simulink model "AD_NOcontrolPIDposicionConObs_CompTermico_rampaPos_EscalVelo"  (R2012b)
settings: Solver=ode45  StartTime=0.0  StopTime=18  MaxStep=1e-4  RelTol=1e-4
values from neighbouring files (symbols this model uses):
  alfa_cu = 3.9*10^-3    (= 0.0039)    [InicializaYconstantes.m]
  b_m = bm+(bl/r^2)    (= 1.5e-05)    [InicializaYconstantes.m]
  Cts = 1.091    [InicializaYconstantes.m]
  J_m = Jm+(Jl/r^2)    (= 5.65099476805e-06)    [InicializaYconstantes.m]
  Kd = J_m*n*wpos    (= 0.0113019895361)    [InicializaYconstantes.m]
  Ketita = 2*3200-b_m/J_m    (= 6397.34560009)    [InicializaYconstantes.m]
  Kew = 3200^2-Ketita*b_m/J_m    (= 10223018.8864)    [InicializaYconstantes.m]
  Ki = J_m*wpos^3    (= 2893.30932124)    [InicializaYconstantes.m]
  Kp = J_m*n*wpos^2    (= 9.04159162887)    [InicializaYconstantes.m]
  lambda = 0.01546    [InicializaYconstantes.m]
  Ld = 6.6*10^-3    (= 0.0066)    [InicializaYconstantes.m]
  Lq = 5.8*10^-3    (= 0.0058)    [InicializaYconstantes.m]
  Pp = 3    [InicializaYconstantes.m]
  r = 314.3008    [InicializaYconstantes.m]
  R1 = -p1i*Lq    (= 29)    [InicializaYconstantes.m]
  R2 = -p1i*Ld    (= 33)    [InicializaYconstantes.m]
  Rs = 1.02    [InicializaYconstantes.m]
  Rs_cero = 1.02    [InicializaYconstantes.m]
  Rts = 55    [InicializaYconstantes.m]
  T_l = Tl/r    (= 0.00499521477515)    [InicializaYconstantes.m]
  Ta = 40    [InicializaYconstantes.m]
undefined symbols (not defined in the file or in its folder): sigbuilder_block
settings Model: Creator=usuario  LastModifiedBy=usuario

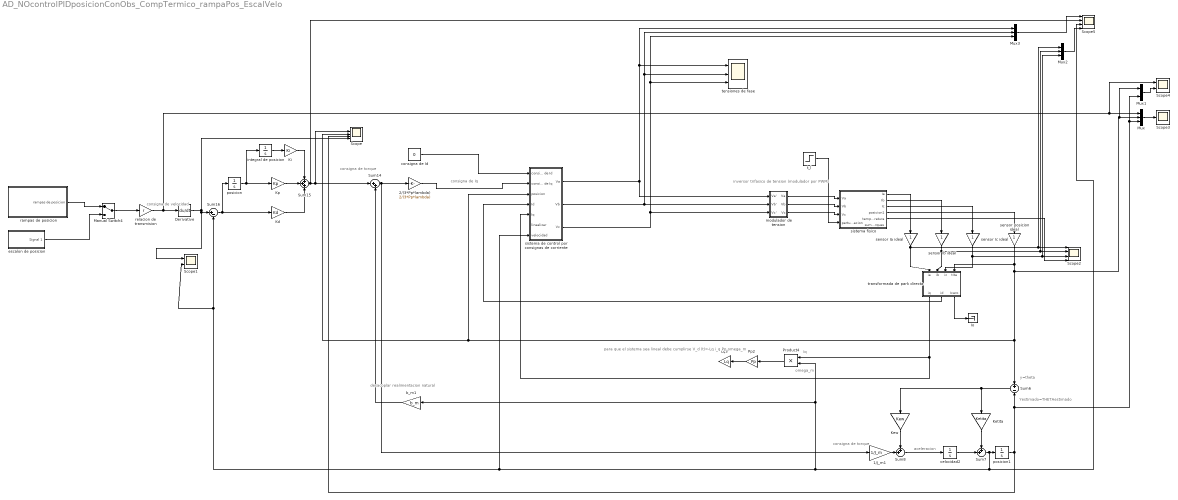
== system AD_NOcontrolPIDposicionConObs_CompTermico_rampaPos_EscalVelo ==
  note: consigna de velocidad
  note: aceleracion
  note: consigna de torque
  note: Yestimado=THETAestimado
  note: y=theta
  note: consigna de torque
  note: desacoplar
      | realimentacion natural
  note: consigna de Iq
  note: inversor trifasico de tension
      | (modulador por PWM)
  note: omega_m
  note: Iq
  note: para que el sistema sea lineal debe cumplirse
      | V_d (t)=-Lq  i_q  Pp omega_m
  1/J_m1 : Gain  Gain=1/J_m
  2/(3*Pp*lambda) : Gain  Gain=2/(3*Pp*lambda)
  Derivative : Derivative
  Io : Terminator
  Kd : Gain  Gain=Kd
  Ketita : Gain  Gain=Ketita
  Kew : Gain  Gain=Kew
  Ki : Gain  Gain=Ki
  Kp : Gain  Gain=Kp
  Lq3 : Gain  Gain=Lq
  Manual Switch4 : ManualSwitch
  Mux : Mux  Inputs=3
  Mux1 : Mux  Inputs=2
  Mux2 : Mux  Inputs=3
  Mux3 : Mux  Inputs=3
  Pp2 : Gain  Gain=Pp
  Product4 : Product  RndMeth=Zero
  Scope : Scope  NumInputPorts=5
      settings: TimeRange=10  YMin=2500~900~-400000~-400000~-2000  YMax=3200~1300~-200000~-200000~2000  SaveName=ScopeData5
  Scope1 : Scope  NumInputPorts=2
      settings: TimeRange=30  YMin=-5~-5.5  YMax=1~1  SaveName=ScopeData7
  Scope2 : Scope  NumInputPorts=4
      settings: YMin=-10~-50~-30~90  YMax=50~20~40~98  SaveName=ScopeData6
  Scope3 : Scope
      settings: TimeRange=10  YMin=-0.5  YMax=6  SaveName=ScopeData8
  Scope4 : Scope  NumInputPorts=2
      settings: TimeRange=10  YMin=-0.5~0  YMax=6~7  SaveName=ScopeData9
  Scope5 : Scope  NumInputPorts=4
      settings: YMin=-0.01~-0.08~-0.075~20  YMax=0.08~0.02~0.075~60  SaveName=ScopeData10
  Sum14 : Sum  Inputs=|++
  Sum15 : Sum  Inputs=+++
  Sum16 : Sum  Inputs=|+-
  Sum6 : Sum  Inputs=+-
  Sum7 : Sum  Inputs=++|
  Sum8 : Sum  Inputs=++|
  b_m1 : Gain  Gain=b_m
  consigna de Id : Constant  Value=0
  escalon de posicion : Subsystem  Tag=STV Subsys  LoadFcn=sigbuilder_block('load');  StartFcn=sigbuilder_block('start');  StopFcn=sigbuilder_block('stop');  ClipboardFcn=sigbuilder_block('clipboard');  mask(Sigbuilder block){}
      mask help: Simulink:masks:SigbuilderBlock_MD
      mask init:
      | if ~strcmp(get_param(bdroot(gcbh),'SimulationStatus'),'stopped') tuvar = sigbuilder_block('maskInit'); end
      settings: CopyFcn=sigbuilder_block('copy');  DeleteFcn=sigbuilder_block('delete');  ModelCloseFcn=sigbuilder_block('modelClose');  PreSaveFcn=sigbuilder_block('preSave');  PauseFcn=sigbuilder_block('pause');  ContinueFcn=sigbuilder_block('continue');  NameChangeFcn=sigbuilder_block('namechange');  OpenFcn=sigbuilder_block('open',[5.58621 27.931 836.69 391.034 ]);  CloseFcn=sigbuilder_block('close');
      mask Display: plot(0, 0, 100, 100,[2, 2, 32, 32, 2], [68, 8, 8, 68, 68],[32, 2], [38, 38], [32, 19, 2],[53, 60, 44], [32, 17, 17, 2],[16, 16, 31, 31]);txt = getActiveGroup(gcbh);text(2, 100, txt,'verticalAlignment', 'top');
  integral de posicion : Integrator
  modulador de tension : Subsystem
  posicion : Integrator
  posicion1 : Integrator
  rampas de posicion : Subsystem  Tag=STV Subsys  LoadFcn=sigbuilder_block('load');  StartFcn=sigbuilder_block('start');  StopFcn=sigbuilder_block('stop');  ClipboardFcn=sigbuilder_block('clipboard');  mask(Sigbuilder block){}
      mask help: Simulink:masks:SigbuilderBlock_MD
      mask init:
      | if ~strcmp(get_param(bdroot(gcbh),'SimulationStatus'),'stopped') tuvar = sigbuilder_block('maskInit'); end
      settings: CopyFcn=sigbuilder_block('copy');  DeleteFcn=sigbuilder_block('delete');  ModelCloseFcn=sigbuilder_block('modelClose');  PreSaveFcn=sigbuilder_block('preSave');  PauseFcn=sigbuilder_block('pause');  ContinueFcn=sigbuilder_block('continue');  NameChangeFcn=sigbuilder_block('namechange');  OpenFcn=sigbuilder_block('open',[5.58621 27.931 836.69 391.034 ]);  CloseFcn=sigbuilder_block('close');
      mask Display: plot(0, 0, 100, 100,[2, 2, 32, 32, 2], [68, 8, 8, 68, 68],[32, 2], [38, 38], [32, 19, 2],[53, 60, 44], [32, 17, 17, 2],[16, 16, 31, 31]);txt = getActiveGroup(gcbh);text(2, 100, txt,'verticalAlignment', 'top');
  "relacion de transmision " : Gain  Gain=r
  sensor Ia ideal : Gain
  sensor Ib ideal : Gain
  sensor Ic ideal : Gain
  sensor posicion ideal : Gain
  sistema de control por consignas de corriente : Subsystem
  sistema fisico : Subsystem
  t_l : Step  Time=1.1  After=T_l  SampleTime=0
  tensiones de fase : Scope  NumInputPorts=3
      settings: TimeRange=8  YMin=-200~-200~-200  YMax=200~200~200  SaveName=ScopeData3  MaxDataPoints=8000
  transformada de park directa : Subsystem
  velocidad2 : Integrator
  wires:
  Ki/1 -> Sum15/1
  Kp/1 -> Sum15/2
  Kd/1 -> Sum15/3
  integral de posicion/1 -> Ki/1
  Sum16/1 -> Kd/1, posicion/1
  sensor Ia ideal/1 -> transformada de park directa/1(ia), Scope2/1, Mux2/1
  sensor Ib ideal/1 -> transformada de park directa/2(ib), Mux2/2, Scope2/2
  sensor Ic ideal/1 -> transformada de park directa/3(ic), Mux2/3, Scope2/3
  Product4/1 -> Pp2/1
  Pp2/1 -> Lq3/1
  modulador de tension/1(Va) -> sistema fisico/1(Va)
  modulador de tension/2(Vb) -> sistema fisico/2(Vb)
  modulador de tension/3(Vc) -> sistema fisico/3(Vc)
  sistema fisico/1(Ia) -> sensor Ia ideal/1
  sistema fisico/2(Ib) -> sensor Ib ideal/1
  sistema fisico/3(Ic) -> sensor Ic ideal/1
  sistema fisico/4(posicion1) -> sensor posicion ideal/1
  transformada de park directa/1(iq) -> sistema de control por consignas de corriente/5(Iq), Product4/1
  transformada de park directa/3(Icero) -> Io/1
  sistema de control por consignas de corriente/1(Va) -> Mux3/1, tensiones de fase/1, modulador de tension/1(Va')
  sistema de control por consignas de corriente/3(Vc) -> Mux3/3, tensiones de fase/3, modulador de tension/3(Vc')
  sistema de control por consignas de corriente/2(Vb) -> modulador de tension/2(Vb'), Mux3/2, tensiones de fase/2
  consigna de Id/1 -> sistema de control por consignas de corriente/1(consigna de Id)
  2/(3*Pp*lambda)/1 -> sistema de control por consignas de corriente/2(consigna de Iq)
  transformada de park directa/2(id) -> sistema de control por consignas de corriente/4(Id)
  b_m1/1 -> Sum14/2
  Sum14/1 -> 2/(3*Pp*lambda)/1, 1/J_m1/1
  Ketita/1 -> Sum7/1
  Kew/1 -> Sum8/1
  1/J_m1/1 -> Sum8/2
  Sum8/1 -> velocidad2/1
  Sum6/1 -> Kew/1, Ketita/1
  posicion/1 -> integral de posicion/1, Kp/1
  velocidad2/1 -> Sum7/2
  sistema fisico/5(temperatura) -> Scope2/4
  Derivative/1 -> Scope1/1, Sum16/1, Scope/5
  sensor posicion ideal/1 -> Sum6/1, sistema de control por consignas de corriente/3(posicion), Scope/3, Mux1/1, Mux/2, transformada de park directa/4(tita)
  posicion1/1 -> Mux1/2, Mux/3, Sum6/2, Scope/4
  Mux/1 -> Scope3/1
  Sum7/1 -> Scope5/3, sistema de control por consignas de corriente/7(velocidad), Scope1/2, Sum16/2, b_m1/1, Product4/2, posicion1/1
  rampas de posicion/1(rampas de posicion) -> Manual Switch4/1
  escalon de posicion/1(Signal 1) -> Manual Switch4/2
  Manual Switch4/1 -> "relacion de transmision "/1
  "relacion de transmision "/1 -> Scope4/1, Mux/1, Derivative/1
  Mux1/1 -> Scope4/2
  t_l/1 -> sistema fisico/4(perturbacion)
  Mux2/1 -> Scope5/4
  Mux3/1 -> Scope5/1
  Sum15/1 -> Sum14/1, Scope/2, Scope5/2

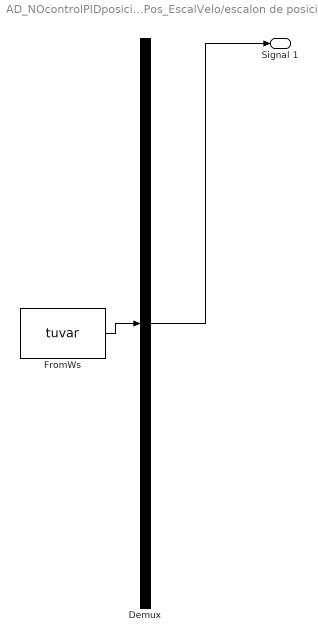
== system AD_NOcontrolPIDposicionConObs_CompTermico_rampaPos_EscalVelo/escalon de posicion ==
  Demux : Demux  Tag=STV Demux  Outputs=1
  FromWs : FromWorkspace  Tag=STV FromWs  VariableName=tuvar  SampleTime=0
      SigBuilderData=|
      | common.afterFinalStr = 'Extrapolate'
      | common.sampleTime = 0
      | dataSet.timeRange = [0 10]
      | dataSet.name = 'Group 1'
      | sbobj.Groups.Name = 'Group 1'
      | sbobj.Groups.Signals.Name = 'Signal 1'
      | sbobj.Groups.Signals.XData = [0 1 1 5 5 10]
      | sbobj.Groups.Signals.YData = [0 0 0.25 0.25 0 0]
  Signal 1 : Outport  Tag=STV Outport
  wires:
  Demux/1 -> Signal 1/1
  FromWs/1 -> Demux/1

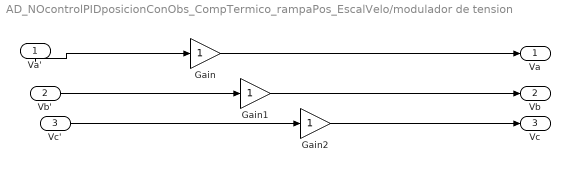
== system AD_NOcontrolPIDposicionConObs_CompTermico_rampaPos_EscalVelo/modulador de tension ==
  Va' : Inport
  Vb' : Inport  Port=2
  Vc' : Inport  Port=3
  Gain : Gain
  Gain1 : Gain
  Gain2 : Gain
  Va : Outport
  Vb : Outport  Port=2
  Vc : Outport  Port=3
  wires:
  Gain/1 -> Va/1
  Gain1/1 -> Vb/1
  Vb'/1 -> Gain1/1
  Va'/1 -> Gain/1
  Vc'/1 -> Gain2/1
  Gain2/1 -> Vc/1

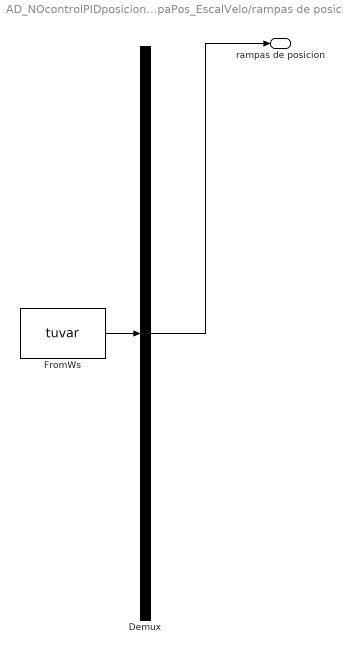
== system AD_NOcontrolPIDposicionConObs_CompTermico_rampaPos_EscalVelo/rampas de posicion ==
  Demux : Demux  Tag=STV Demux  Outputs=1
  FromWs : FromWorkspace  Tag=STV FromWs  VariableName=tuvar  SampleTime=0
      SigBuilderData=|
      | common.afterFinalStr = 'Extrapolate'
      | common.sampleTime = 0
      | dataSet.timeRange = [0 30]
      | dataSet.name = 'Group 1'
      | sbobj.Groups.Name = 'Group 1'
      | sbobj.Groups.Signals.Name = 'rampas de posicion'
      | sbobj.Groups.Signals.XData = [0 1 6 11 16 30]
      | sbobj.Groups.Signals.YData = [0 0 6.28318530718 6.28318530718 0 0]
      | sbobj.Groups.TimeRange = [0 30]
  rampas de posicion : Outport  Tag=STV Outport
  wires:
  Demux/1 -> rampas de posicion/1
  FromWs/1 -> Demux/1

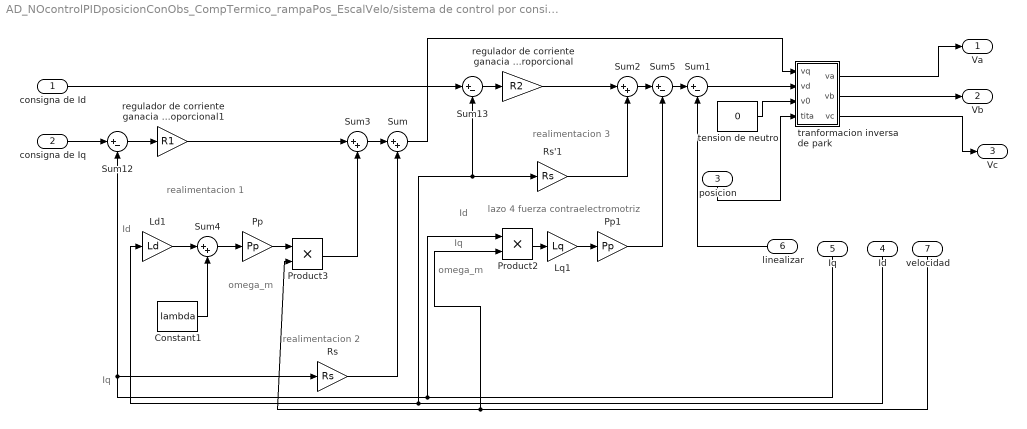
== system AD_NOcontrolPIDposicionConObs_CompTermico_rampaPos_EscalVelo/sistema de control por consignas de corriente ==
  note: Id
  note: realimentacion 3
  note: Iq
  note: realimentacion 1
  note: Id
  note: omega_m
  note: realimentacion 2
  note: lazo 4 fuerza contraelectromotriz
  note: omega_m
  note: Iq
  consigna de Id : Inport
  consigna de Iq : Inport  Port=2
  posicion : Inport  Port=3
  Id : Inport  Port=4
  Iq : Inport  Port=5
  linealizar : Inport  Port=6
  velocidad : Inport  Port=7
  Constant1 : Constant  Value=lambda
  Ld1 : Gain  Gain=Ld
  Lq1 : Gain  Gain=Lq
  Pp : Gain  Gain=Pp
  Pp1 : Gain  Gain=Pp
  Product2 : Product  RndMeth=Zero
  Product3 : Product  RndMeth=Zero
  Rs : Gain  Gain=Rs
  Rs'1 : Gain  Gain=Rs
  Sum{,2..4} (4 alike) : Sum  Inputs=|++
  Sum{1,5,12..13} (4 alike) : Sum  Inputs=|+-
  regulador de corriente ganacia proporcional : Gain  Gain=R2
  regulador de corriente ganacia proporcional1 : Gain  Gain=R1
  tension de neutro : Constant  Value=0
  tranformacion inversa de park : Subsystem
  Va : Outport
  Vb : Outport  Port=2
  Vc : Outport  Port=3
  wires:
  regulador de corriente ganacia proporcional1/1 -> Sum3/1
  tension de neutro/1 -> tranformacion inversa de park/3(v0)
  Rs/1 -> Sum/2
  Sum4/1 -> Pp/1
  Constant1/1 -> Sum4/2
  Sum12/1 -> regulador de corriente ganacia proporcional1/1
  linealizar/1 -> Sum1/2
  Sum1/1 -> tranformacion inversa de park/2(vd)
  tranformacion inversa de park/1(va) -> Va/1
  tranformacion inversa de park/3(vc) -> Vc/1
  Ld1/1 -> Sum4/1
  Sum/1 -> tranformacion inversa de park/1(vq)
  Id/1 -> Ld1/1, Sum13/2, Rs'1/1
  Pp/1 -> Product3/1
  regulador de corriente ganacia proporcional/1 -> Sum2/1
  consigna de Id/1 -> Sum13/1
  Rs'1/1 -> Sum2/2
  consigna de Iq/1 -> Sum12/1
  tranformacion inversa de park/2(vb) -> Vb/1
  Sum13/1 -> regulador de corriente ganacia proporcional/1
  Product3/1 -> Sum3/2
  Sum3/1 -> Sum/1
  posicion/1 -> tranformacion inversa de park/4(tita)
  Product2/1 -> Lq1/1
  Iq/1 -> Rs/1, Sum12/2, Product2/1
  Lq1/1 -> Pp1/1
  Pp1/1 -> Sum5/2
  velocidad/1 -> Product3/2, Product2/2
  Sum5/1 -> Sum1/1
  Sum2/1 -> Sum5/1

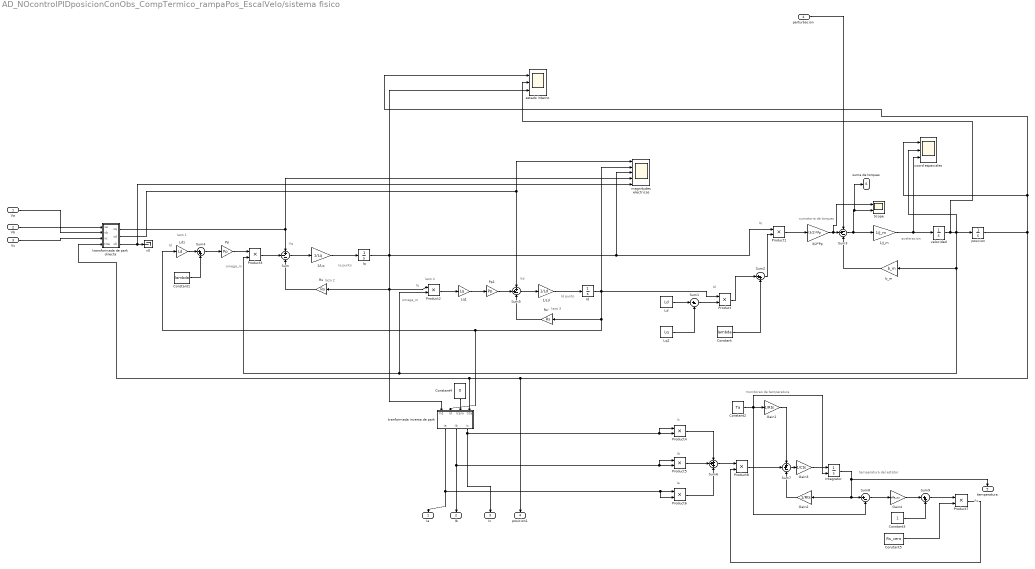
== system AD_NOcontrolPIDposicionConObs_CompTermico_rampaPos_EscalVelo/sistema fisico ==
  note: Rs
  note: lazo 4
  note: lazo 3
  note: lazo 2
  note: lazo 1
  note: sumatoria de torques
  note: Vd
  note: omega_m
  note: Iq
  note: Id punto
  note: Vq
  note: Id
  note: Iq punto
  note: Iq
  note: aceleracion
  note: Id
  note: omega_m
  note: monitoreo de temperatura
  note: temperatura del estator
  note: Ic
  note: Ib
  note: Ia
  Va : Inport
  Vb : Inport  Port=2
  Vc : Inport  Port=3
  perturbacion : Inport  Port=4
  1/J_m : Gain  Gain=1/J_m
  1/Ld : Gain  Gain=1/Ld
  1/Lq : Gain  Gain=1/Lq
  3/2*Pp : Gain  Gain=(3/2)*Pp
  Constant : Constant  Value=lambda
  Constant1 : Constant  Value=lambda
  Constant2 : Constant  Value=Ta
  Constant3 : Constant
  Constant4 : Constant  Value=0
  Constant5 : Constant  Value=Rs_cero
  Gain1 : Gain  Gain=1/Rts
  Gain2 : Gain  Gain=1/Rts
  Gain3 : Gain  Gain=1/Cts
  Gain4 : Gain  Gain=alfa_cu
  Id : Integrator
  Integrator : Integrator  InitialConditionSource=external
  Iq : Integrator
  Ld : Constant  Value=Ld
  Ld1 : Gain  Gain=Ld
  Lq1 : Gain  Gain=Lq
  Lq2 : Constant  Value=Lq
  Pp : Gain  Gain=Pp
  Pp1 : Gain  Gain=Pp
  Product{,1..8} (9 alike) : Product  RndMeth=Zero
  Rs : Gain  Gain=Rs
  Rs' : Gain  Gain=Rs
  Scope : Scope  NumInputPorts=2
      settings: YMin=-5~-5  YMax=5~5  SaveName=ScopeData4
  Sum : Sum  Inputs=+--
  Sum1 : Sum  Inputs=|+-
  Sum2 : Sum  Inputs=|++
  Sum3 : Sum  Inputs=-+-
  Sum4 : Sum  Inputs=|++
  Sum5 : Sum  Inputs=++-
  Sum6 : Sum  Inputs=+++
  Sum7 : Sum  Inputs=++-
  Sum8 : Sum  Inputs=|+-
  Sum9 : Sum  Inputs=|++
  b_m : Gain  Gain=b_m
  coord espaciales : Scope  NumInputPorts=3
      settings: TimeRange=12  YMin=-1000~0~-50000  YMax=3000~300~100000  MaxDataPoints=8000
  estado interno : Scope  NumInputPorts=3
      settings: TimeRange=10  YMin=-2000~0~-5  YMax=6000~600~10  MaxDataPoints=8000
  magnitudes electricas : Scope  NumInputPorts=5
      settings: TimeRange=10  YMin=-0.2~-1~-0.05~-10~-1  YMax=0.2~1~0.05~0~1  SaveName=ScopeData2  MaxDataPoints=8000
  posicion : Integrator
  "tranformada inversa de park " : Subsystem
  transformada de park directa : Subsystem
  v0 : Terminator
  velocidad : Integrator  ContinuousStateAttributes='velocidad'
  Ia : Outport
  Ib : Outport  Port=2
  Ic : Outport  Port=3
  posicion1 : Outport  Port=4
  temperatura : Outport  Port=5
  suma de torques : Outport  Port=6
  wires:
  Product/1 -> Sum2/1
  Ld/1 -> Sum1/1
  Lq2/1 -> Sum1/2
  Sum1/1 -> Product/2
  Constant/1 -> Sum2/2
  Sum2/1 -> Product1/2
  1/Lq/1 -> Iq/1
  Product1/1 -> 3/2*Pp/1
  Ld1/1 -> Sum4/1
  Sum3/1 -> Scope/2, suma de torques/1, 1/J_m/1
  1/Ld/1 -> Id/1
  Constant1/1 -> Sum4/2
  b_m/1 -> Sum3/3
  Sum4/1 -> Pp/1
  Sum/1 -> 1/Lq/1
  Rs/1 -> Sum/3
  perturbacion/1 -> Sum3/1
  Rs'/1 -> Sum5/3
  Product2/1 -> Lq1/1
  Iq/1 -> estado interno/3, magnitudes electricas/3, Product1/1, "tranformada inversa de park "/1(In1), Rs/1, Product2/1
  Lq1/1 -> Pp1/1
  Product3/1 -> Sum/2
  transformada de park directa/1(vq) -> magnitudes electricas/4, Sum/1
  transformada de park directa/2(vd) -> magnitudes electricas/1, Sum5/1
  Sum5/1 -> 1/Ld/1
  3/2*Pp/1 -> Scope/1, Sum3/2
  1/J_m/1 -> coord espaciales/3, velocidad/1
  Pp1/1 -> Sum5/2
  transformada de park directa/3(v0) -> magnitudes electricas/5, v0/1
  posicion/1 -> transformada de park directa/4(tita), "tranformada inversa de park "/4(tita), posicion1/1, estado interno/1, coord espaciales/1
  velocidad/1 -> coord espaciales/2, Product2/2, Product3/2, b_m/1, posicion/1, estado interno/2
  Pp/1 -> Product3/1
  Id/1 -> "tranformada inversa de park "/2(Id), Ld1/1, Rs'/1, Product/1, magnitudes electricas/2
  Constant4/1 -> "tranformada inversa de park "/3(Icero)
  Vc/1 -> transformada de park directa/3(vc)
  Vb/1 -> transformada de park directa/2(vb)
  Va/1 -> transformada de park directa/1(va)
  "tranformada inversa de park "/1(ia) -> Ia/1, Product6/2, Product6/1
  "tranformada inversa de park "/2(ib) -> Ib/1, Product5/2, Product5/1
  "tranformada inversa de park "/3(ic) -> Ic/1, Product4/1, Product4/2
  Product4/1 -> Sum6/1
  Product5/1 -> Sum6/2
  Product6/1 -> Sum6/3
  Product8/1 -> Sum7/2
  Constant2/1 -> Sum8/2, Gain1/1, Integrator/2
  Gain1/1 -> Sum7/1
  Sum7/1 -> Gain3/1
  Gain3/1 -> Integrator/1
  Integrator/1 -> temperatura/1, Sum8/1, Gain2/1
  Gain2/1 -> Sum7/3
  Sum8/1 -> Gain4/1
  Gain4/1 -> Sum9/1
  Constant3/1 -> Sum9/2
  Sum9/1 -> Product7/1
  Constant5/1 -> Product7/2
  Product7/1 -> Product8/2
  Sum6/1 -> Product8/1

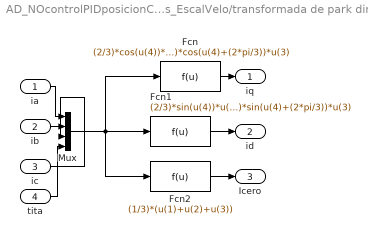
== system AD_NOcontrolPIDposicionConObs_CompTermico_rampaPos_EscalVelo/transformada de park directa ==
  ia : Inport
  ib : Inport  Port=2
  ic : Inport  Port=3
  tita : Inport  Port=4
  Fcn : Fcn  Expr=(2/3)*cos(u(4))*u(1)+(2/3)*cos(u(4)-(2*pi/3))*u(2)+(2/3)*cos(u(4)+(2*pi/3))*u(3)
  Fcn1 : Fcn  Expr=(2/3)*sin(u(4))*u(1)+(2/3)*sin(u(4)-(2*pi/3))*u(2)+(2/3)*sin(u(4)+(2*pi/3))*u(3)
  Fcn2 : Fcn  Expr=(1/3)*(u(1)+u(2)+u(3))
  Mux : Mux
  iq : Outport
  id : Outport  Port=2
  Icero : Outport  Port=3
  wires:
  Mux/1 -> Fcn1/1, Fcn/1, Fcn2/1
  Fcn/1 -> iq/1
  ia/1 -> Mux/1
  ib/1 -> Mux/2
  Fcn1/1 -> id/1
  ic/1 -> Mux/3
  tita/1 -> Mux/4
  Fcn2/1 -> Icero/1

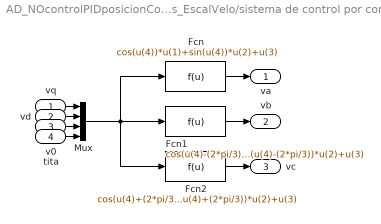
== system AD_NOcontrolPIDposicionConObs_CompTermico_rampaPos_EscalVelo/sistema de control por consignas de corriente/tranformacion inversa de park ==
  vq : Inport
  vd : Inport  Port=2
  v0 : Inport  Port=3
  tita : Inport  Port=4
  Fcn : Fcn  Expr=cos(u(4))*u(1)+sin(u(4))*u(2)+u(3)
  Fcn1 : Fcn  Expr=cos(u(4)-(2*pi/3))*u(1)+sin(u(4)-(2*pi/3))*u(2)+u(3)
  Fcn2 : Fcn  Expr=cos(u(4)+(2*pi/3))*u(1)+sin(u(4)+(2*pi/3))*u(2)+u(3)
  Mux : Mux
  va : Outport
  vb : Outport  Port=2
  vc : Outport  Port=3
  wires:
  Mux/1 -> Fcn1/1, Fcn/1, Fcn2/1
  Fcn/1 -> va/1
  vq/1 -> Mux/1
  vd/1 -> Mux/2
  Fcn1/1 -> vb/1
  v0/1 -> Mux/3
  tita/1 -> Mux/4
  Fcn2/1 -> vc/1

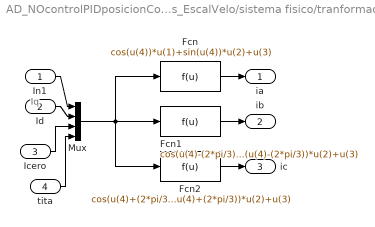
== system AD_NOcontrolPIDposicionConObs_CompTermico_rampaPos_EscalVelo/sistema fisico/tranformada inversa de park  ==
  note: Iq
  In1 : Inport
  Id : Inport  Port=2
  Icero : Inport  Port=3
  tita : Inport  Port=4
  Fcn : Fcn  Expr=cos(u(4))*u(1)+sin(u(4))*u(2)+u(3)
  Fcn1 : Fcn  Expr=cos(u(4)-(2*pi/3))*u(1)+sin(u(4)-(2*pi/3))*u(2)+u(3)
  Fcn2 : Fcn  Expr=cos(u(4)+(2*pi/3))*u(1)+sin(u(4)+(2*pi/3))*u(2)+u(3)
  Mux : Mux
  ia : Outport
  ib : Outport  Port=2
  ic : Outport  Port=3
  wires:
  Mux/1 -> Fcn1/1, Fcn/1, Fcn2/1
  Fcn/1 -> ia/1
  In1/1 -> Mux/1
  Id/1 -> Mux/2
  Fcn1/1 -> ib/1
  Icero/1 -> Mux/3
  tita/1 -> Mux/4
  Fcn2/1 -> ic/1

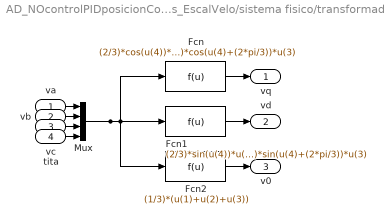
== system AD_NOcontrolPIDposicionConObs_CompTermico_rampaPos_EscalVelo/sistema fisico/transformada de park directa ==
  va : Inport
  vb : Inport  Port=2
  vc : Inport  Port=3
  tita : Inport  Port=4
  Fcn : Fcn  Expr=(2/3)*cos(u(4))*u(1)+(2/3)*cos(u(4)-(2*pi/3))*u(2)+(2/3)*cos(u(4)+(2*pi/3))*u(3)
  Fcn1 : Fcn  Expr=(2/3)*sin(u(4))*u(1)+(2/3)*sin(u(4)-(2*pi/3))*u(2)+(2/3)*sin(u(4)+(2*pi/3))*u(3)
  Fcn2 : Fcn  Expr=(1/3)*(u(1)+u(2)+u(3))
  Mux : Mux
  vq : Outport
  vd : Outport  Port=2
  v0 : Outport  Port=3
  wires:
  Mux/1 -> Fcn1/1, Fcn/1, Fcn2/1
  Fcn/1 -> vq/1
  va/1 -> Mux/1
  vb/1 -> Mux/2
  Fcn1/1 -> vd/1
  vc/1 -> Mux/3
  tita/1 -> Mux/4
  Fcn2/1 -> v0/1
